simulink model "SPWM_tiaozhi_simscape"  (R2026a)
settings: Solver=ode23t  StartTime=1  StopTime=20  RelTol=1e-5  AbsTol=1e-5
undefined symbols (not defined in the file): PermanentMagnetSynchrono_class
libraries: fl_lib x21, nesl_utility x18, ee_lib x7, eeTransforms x2, elec_conv_HighZElecRef x1, simulink x1
settings Model: SimulationMode=accelerator  Creator=刘炳宏  LastModifiedBy=mushen
settings DebuggingCC: SaveWithParameterizedLinksMsg=none
settings SimscapeCC: SimscapeLogType=none  SimscapeLogDataHistory=5000.0

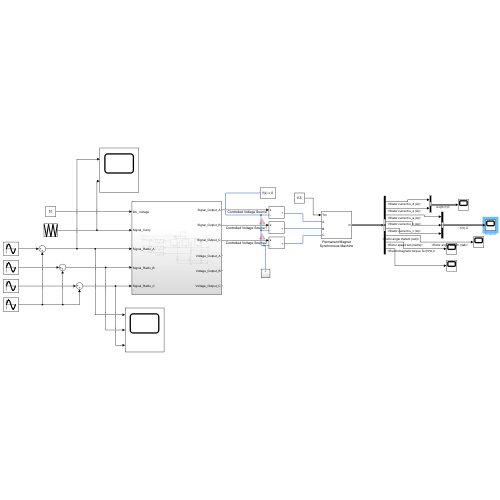
[thumbnail: Simulink's stored preview of the top-level diagram]
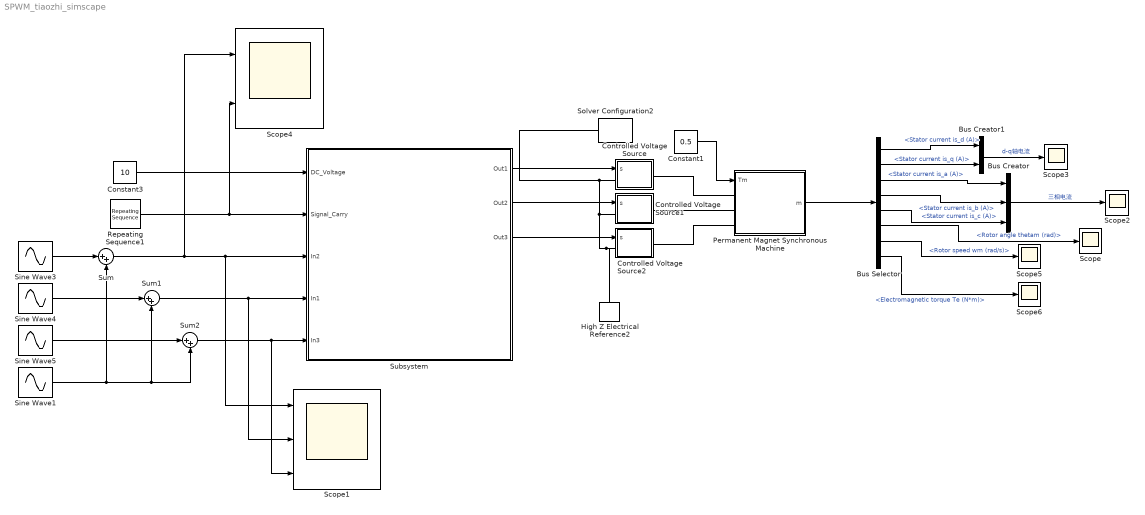
== system SPWM_tiaozhi_simscape ==
  Bus Creator : BusCreator  Inputs=3
  Bus Creator1 : BusCreator  Inputs=2
  Bus Selector : BusSelector  OutputSignals=Stator current is_d (A),Stator current is_q (A),Stator current is_a (A),Stator current is_b (A),Stator current is_c (A),Rotor angle thetam (rad),Rotor speed wm (rad/s),Electromagnetic torque Te (N*m)
  Constant1 : Constant  Value=0.5
  Constant3 : Constant  Value=10
  Controlled Voltage Source : Subsystem
      settings: OpenFcn=elec.conv.unmask(gcb);
  Controlled Voltage Source1 : Subsystem
      settings: OpenFcn=elec.conv.unmask(gcb);
  Controlled Voltage Source2 : Subsystem
      settings: OpenFcn=elec.conv.unmask(gcb);
  High Z Electrical Reference2 : elec_conv_HighZElecRef/High Z Electrical Reference  SystemSampleTime=-1  VariantActivationTime=update diagram  EmptyChoice=off  PassThrough=off  PassThroughVariantControl=(default)  EmptyChoiceVariantControl=(default)  AllowFlexibleInterface=on  Latency=0  AutoFrameSizeCalculation=off
  Permanent Magnet Synchronous Machine : Subsystem
      settings: OpenFcn=elec.conv.unmask(gcb);
  Repeating Sequence1 : simulink/Sources/Repeating Sequence  rep_seq_t=[0,0.5/(5000),1/(5000)]  rep_seq_y=[1,-1,1]
  Scope{,2..3,5..6} (5 alike) : Scope
      Scope settings: ActiveDisplayYMinimum=-0.44345  ActiveDisplayYMaximum=0.09536
      Scope2 settings: ActiveDisplayYMinimum=-3.3210941961077998  ActiveDisplayYMaximum=2.6978662354691325  DataLoggingVariableName=ScopeData2
      Scope3 settings: ActiveDisplayYMinimum=-2.66955  ActiveDisplayYMaximum=3.4348
      Scope5 settings: ActiveDisplayYMinimum=-16.20295  ActiveDisplayYMaximum=14.7299  DataLoggingVariableName=ScopeData3
      Scope6 settings: ActiveDisplayYMinimum=-7.90574  ActiveDisplayYMaximum=7.97374  DataLoggingVariableName=ScopeData4
  Scope1 : Scope  NumInputPorts=3
      settings: SampleTime=0.0000  ActiveDisplayYMinimum=-0.62058705897297939  ActiveDisplayYMaximum=0.62058707725034468  DataLoggingVariableName=Ratio
  Scope4 : Scope  NumInputPorts=2
      settings: SampleTime=0.0000  ActiveDisplayYMinimum=-1.25  ActiveDisplayYMaximum=1.25  DataLoggingVariableName=Ratio1
  Sine Wave1 : Sin  Amplitude=0.02*10  Frequency=6*3.14159*5*10  SampleTime=0
  Sine Wave3 : Sin  Amplitude=0.05*10  Frequency=2*3.14159*5*10  SampleTime=0
  Sine Wave4 : Sin  Amplitude=0.05*10  Frequency=2*3.14159*5*10  Phase=2*3.14159/3  SampleTime=0
  Sine Wave5 : Sin  Amplitude=0.05*10  Frequency=2*3.14159*5*10  Phase=-2*3.14159/3  SampleTime=0
  Solver Configuration2 : nesl_utility/Solver Configuration  PhysicalDomain=network_engine_domain  SubClassName=solver  LeftPortType=input  RightPortType=generic  Tones=[]  Harmonics=[]  SimulateNoise=off  Profile=off  UseLocalSampling=off  EnableSwitchedLinearOptims=on  FrequencyDomain=off  UseCCode=off  RelTol=0.001  AbsTol=0.001  MinStep=1e-09  ToWorkspace=off  RevertToSquareIcSolve=off  NumHomotopyIterations=100  PhasorMode=off  PhasorModeNumHarmonics=1  ConsistencySolver=NEWTON_XTOL_AFTER_FTOL  CanonicalOrdering=UNORDERED  OptimizeIntermediates=UNOPTIMIZED  IndexReductionMethod=DerivativeReplacement  DoDC=off  ResidualTolerance=1e-09  ConsistencyTolSource=GLOBAL  ConsistencyAbsTol=0.001  ConsistencyRelTol=0.001  ConsistencyTolFactor=0.001  UseLocalSolver=off  LocalSolverChoice=NE_BACKWARD_EULER_ADVANCER  ResolveIndetEquations=on  FunctionEvalNumThread=1  LocalSolverSampleTime=0.001  DoFixedCost=off  MaxNonlinIter=3  MaxModeIter=2  ComputeImpulses=off  ImpulseIterations=2  LinearAlgebra=auto  LinearAlgebraNumThread=0  EquationFormulation=NE_TIME_EF  DelaysMemoryBudget=1024  AutomaticFiltering=on  FilteringTimeConstant=0.001  PartitionStorageMethod=AS_NEEDED  PartitionMemoryBudget=1024  PartitionMethod=ROBUST  MultibodyUseLocalSolver=off  MultibodyLocalSolverChoice=ODE1  MultibodyLocalSolverSampleTime=0.001
  Subsystem : Subsystem
  Sum : Sum  Inputs=|++
  Sum1 : Sum  Inputs=|++
  Sum2 : Sum  Inputs=|++
  wires:
  Repeating Sequence1/1 -> Scope4/2, Subsystem/2(Signal_Carry)
  Constant3/1 -> Subsystem/1(DC_Voltage)
  Sine Wave3/1 -> Sum/1
  Sum/1 -> Scope4/1, Scope1/1, Subsystem/3(In2)
  Sum1/1 -> Scope1/2, Subsystem/4(In1)
  Sine Wave4/1 -> Sum1/1
  Sine Wave1/1 -> Sum2/2, Sum1/2, Sum/2
  Sine Wave5/1 -> Sum2/1
  Sum2/1 -> Scope1/3, Subsystem/5(In3)
  Subsystem/1(Out1) -> Controlled Voltage Source/1(s)
  Subsystem/3(Out3) -> Controlled Voltage Source2/1(s)
  Subsystem/2(Out2) -> Controlled Voltage Source1/1(s)
  Bus Selector/5 -> Bus Creator/3  "<Stator current is_c (A)>"
  Bus Selector/4 -> Bus Creator/2  "<Stator current is_b (A)>"
  Bus Selector/2 -> Bus Creator1/2  "<Stator current is_q (A)>"
  Bus Selector/1 -> Bus Creator1/1  "<Stator current is_d (A)>"
  Bus Creator1/1 -> Scope3/1  "d-q轴电流"
  Permanent Magnet Synchronous Machine/1(m) -> Bus Selector/1
  Bus Creator/1 -> Scope2/1  "三相电流"
  Bus Selector/3 -> Bus Creator/1  "<Stator current is_a (A)>"
  Bus Selector/6 -> Scope/1  "<Rotor angle thetam (rad)>"
  Bus Selector/7 -> Scope5/1  "<Rotor speed wm (rad/s)>"
  Bus Selector/8 -> Scope6/1  "<Electromagnetic torque Te (N*m)>"
  Constant1/1 -> Permanent Magnet Synchronous Machine/1(Tm)
  connections:
  Controlled Voltage Source/LConn1 -- Solver Configuration2/RConn1 -- Controlled Voltage Source1/LConn1 -- Controlled Voltage Source2/LConn1 -- High Z Electrical Reference2/LConn1
  Permanent Magnet Synchronous Machine/LConn2 -- Controlled Voltage Source1/RConn1
  Permanent Magnet Synchronous Machine/LConn1 -- Controlled Voltage Source/RConn1
  Permanent Magnet Synchronous Machine/LConn3 -- Controlled Voltage Source2/RConn1

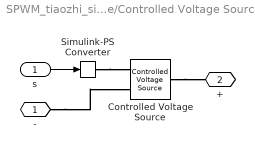
== system SPWM_tiaozhi_simscape/Controlled Voltage Source ==
  s : Inport
  Controlled Voltage Source : fl_lib/Electrical/Electrical Sources/Controlled Voltage Source
  Simulink-PS Converter : nesl_utility/Simulink-PS Converter  PhysicalDomain=network_engine_domain  SubClassName=ps_input  LeftPortType=input  RightPortType=output  PseudoPeriodic=off  Frequencies=[]  NoiseDistribution=none  NoiseParameters=[]  Unit=1  AffineConversion=off  FilteringAndDerivatives=provide  SimscapeFilterOrder=1  InputFilterTimeConstant=0.001  UdotUserProvided=0
  - : PMIOPort  Side=Left
  + : PMIOPort  Port=2  Side=Right
  wires:
  s/1 -> Simulink-PS Converter/1
  connections:
  -/RConn1 -- Controlled Voltage Source/RConn2
  Simulink-PS Converter/RConn1 -- Controlled Voltage Source/RConn1
  Controlled Voltage Source/LConn1 -- +/RConn1

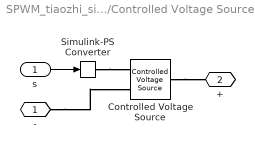
== system SPWM_tiaozhi_simscape/Controlled Voltage Source1 ==
  s : Inport
  Controlled Voltage Source : fl_lib/Electrical/Electrical Sources/Controlled Voltage Source
  Simulink-PS Converter : nesl_utility/Simulink-PS Converter  PhysicalDomain=network_engine_domain  SubClassName=ps_input  LeftPortType=input  RightPortType=output  PseudoPeriodic=off  Frequencies=[]  NoiseDistribution=none  NoiseParameters=[]  Unit=1  AffineConversion=off  FilteringAndDerivatives=provide  SimscapeFilterOrder=1  InputFilterTimeConstant=0.001  UdotUserProvided=0
  - : PMIOPort  Side=Left
  + : PMIOPort  Port=2  Side=Right
  wires:
  s/1 -> Simulink-PS Converter/1
  connections:
  -/RConn1 -- Controlled Voltage Source/RConn2
  Simulink-PS Converter/RConn1 -- Controlled Voltage Source/RConn1
  Controlled Voltage Source/LConn1 -- +/RConn1

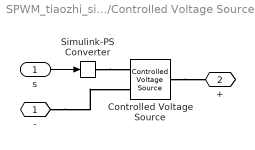
== system SPWM_tiaozhi_simscape/Controlled Voltage Source2 ==
  s : Inport
  Controlled Voltage Source : fl_lib/Electrical/Electrical Sources/Controlled Voltage Source
  Simulink-PS Converter : nesl_utility/Simulink-PS Converter  PhysicalDomain=network_engine_domain  SubClassName=ps_input  LeftPortType=input  RightPortType=output  PseudoPeriodic=off  Frequencies=[]  NoiseDistribution=none  NoiseParameters=[]  Unit=1  AffineConversion=off  FilteringAndDerivatives=provide  SimscapeFilterOrder=1  InputFilterTimeConstant=0.001  UdotUserProvided=0
  - : PMIOPort  Side=Left
  + : PMIOPort  Port=2  Side=Right
  wires:
  s/1 -> Simulink-PS Converter/1
  connections:
  -/RConn1 -- Controlled Voltage Source/RConn2
  Simulink-PS Converter/RConn1 -- Controlled Voltage Source/RConn1
  Controlled Voltage Source/LConn1 -- +/RConn1

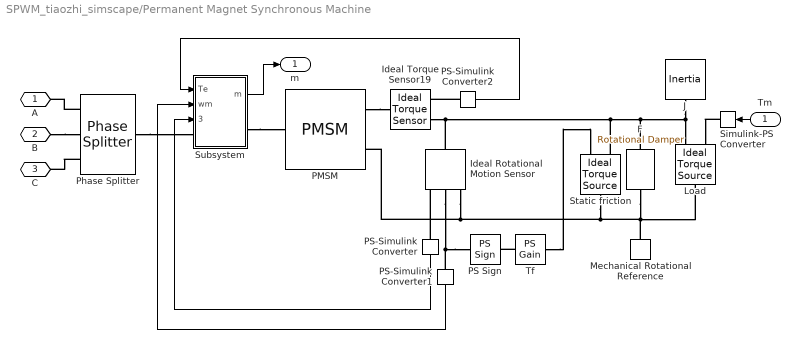
== system SPWM_tiaozhi_simscape/Permanent Magnet Synchronous Machine ==
  Tm : Inport
  F : fl_lib/Mechanical/Rotational Elements/Rotational Damper  D=0.0003505 N*m/(rad/s)  w_specify=on  w_priority=High  w=0 rad/s  w_nominal_specify=off  w_nominal_value=1  w_nominal_unit=rad/s  t_specify=off  t_priority=None  t=0 N*m  t_nominal_specify=off  t_nominal_value=1  t_nominal_unit=N*m
  Ideal Rotational Motion Sensor : fl_lib/Mechanical/Mechanical Sensors/Ideal Rotational Motion Sensor  reference=foundation.enum.MeasurementReference.difference  acceleration_port=false  velocity_port=true  position_port=true  wrap_angle=simscape.enum.onoff.off  offset=1 deg
  Ideal Torque Sensor19 : fl_lib/Mechanical/Mechanical Sensors/Ideal Torque Sensor
  J : fl_lib/Mechanical/Rotational Elements/Inertia  inertia=0.00062 kg*m^2  num_ports=foundation.enum.numPorts2.one  w_specify=on  w_priority=High  w=0 rad/s  w_nominal_specify=off  w_nominal_value=1  w_nominal_unit=rad/s  t_specify=off  t_priority=None  t=0 N*m  t_nominal_specify=off  t_nominal_value=1  t_nominal_unit=N*m
  Load : fl_lib/Mechanical/Mechanical Sources/Ideal Torque Source
  Mechanical Rotational Reference : fl_lib/Mechanical/Rotational Elements/Mechanical Rotational Reference
  PMSM : ee_lib/Electromechanical/Permanent Magnet/PMSM  port_option=ee.enum.threePhasePort.composite  winding_type=ee.enum.statorconnection.wye  machine_param=ee.enum.pmsm.parameterization.constant  nPolePairs=10  pmflux_param=1  pm_flux_linkage=PermanentMagnetSynchrono_class('Torque Tm',[0.00062 0.0003505 10 0],4,'Flux linkage established by magnets (V.s)',0.074147,134.4878,1.1122,'Aligned with phase A axis (original Park)',[0 1 0 0],'Sinusoidal',120,'3',[0 0 0 0 0 0]).objParamMappingDerived.NewDerivedParam.pm_flux_linkage Wb  torque_constant=0.18 N*m/A  back_emf_constant=0.18 V/(rad/s)  stator_param=1  Ld=0.0085 H  Lq=0.0085 H  idVec=[-200, 0, 200] A  iqVec=[-200, 0, 200] A  LdMatrix=0.0002 * ones(3, 3) H  LqMatrix=0.0002 * ones(3, 3) H  PmMatrix=0.1 * ones(3, 3) Wb  ktMatrix=0.18 * ones(3, 3) N*m/A  keMatrix=0.18 * ones(3, 3) V/(rad/s)  L0=1e-09 H  Ls=0.0002 H  Lm=-0.00002 H  Ms=0.00002 H  Rs=0.18 Ohm  zero_sequence=0  axes_param=2  loss_param=ee.enum.ironloss.none  losses_oc=[0, 0, 0] W  losses_sc=[0, 0, 0] W  f_losses=60 Hz  Isc_losses=95 A  J=0 kg*m^2  lam=0 N*m/(rad/s)  i_d_specify=on  i_d_priority=High  i_d=PermanentMagnetSynchrono_class('Torque Tm',[0.00062 0.0003505 10 0],4,'Flux linkage established by magnets (V.s)',0.074147,134.4878,1.1122,'Aligned with phase A axis (original Park)',[0 1 0 0],'Sinusoidal',120,'3',[0 0 0 0 0 0]).objParamMappingDerived.NewDerivedParam.i_d A  i_d_nominal_specify=off  i_d_nominal_value=1  i_d_nominal_unit=A  i_q_specify=on  i_q_priority=High  i_q=PermanentMagnetSynchrono_class('Torque Tm',[0.00062 0.0003505 10 0],4,'Flux linkage established by magnets (V.s)',0.074147,134.4878,1.1122,'Aligned with phase A axis (original Park)',[0 1 0 0],'Sinusoidal',120,'3',[0 0 0 0 0 0]).objParamMappingDerived.NewDerivedParam.i_q A  i_q_nominal_specify=off  i_q_nominal_value=1  i_q_nominal_unit=A  torque_specify=off  torque_priority=None  torque=0 N*m  torque_nominal_specify=off  torque_nominal_value=1  torque_nominal_unit=N*m  angular_velocity_specify=on  angular_velocity_priority=High  angular_velocity=0 rad/s  angular_velocity_nominal_specify=off  angular_velocity_nominal_value=1  angular_velocity_nominal_unit=rpm  angular_position_specify=on  angular_position_priority=High  angular_position=1 deg  angular_position_nominal_specify=off  angular_position_nominal_value=1  angular_position_nominal_unit=deg  alpha=3.93e-3 1/K  alpha_flux=-0.001 1/K  Tmeas=298.15 K  stator_thermal_mass=100 J/K  rotor_thermal_mass=200 J/K  Rm_percent_rotor=90  Rd_percent_rotor=30  temperatureA_specify=off  temperatureA_priority=High  temperatureA=25 degC  temperatureA_nominal_specify=off  temperatureA_nominal_value=1  temperatureA_nominal_unit=degC  temperatureB_specify=off  temperatureB_priority=High  temperatureB=25 degC  temperatureB_nominal_specify=off  temperatureB_nominal_value=1  temperatureB_nominal_unit=degC  temperatureC_specify=off  temperatureC_priority=High  temperatureC=25 degC  temperatureC_nominal_specify=off  temperatureC_nominal_value=1  temperatureC_nominal_unit=degC  temperatureR_specify=off  temperatureR_priority=High  temperatureR=25 degC  temperatureR_nominal_specify=off  temperatureR_nominal_value=1  temperatureR_nominal_unit=degC
  PS Sign : fl_lib/Physical Signals/Nonlinear Operators/PS Sign
  PS-Simulink Converter : nesl_utility/PS-Simulink Converter  PhysicalDomain=network_engine_domain  SubClassName=ps_output  LeftPortType=input  RightPortType=output  PseudoPeriodic=off  Frequencies=[]  VectorFormat=1-D array  Unit=1  AffineConversion=off
  PS-Simulink Converter1 : nesl_utility/PS-Simulink Converter  PhysicalDomain=network_engine_domain  SubClassName=ps_output  LeftPortType=input  RightPortType=output  PseudoPeriodic=off  Frequencies=[]  VectorFormat=1-D array  Unit=1  AffineConversion=off
  PS-Simulink Converter2 : nesl_utility/PS-Simulink Converter  PhysicalDomain=network_engine_domain  SubClassName=ps_output  LeftPortType=input  RightPortType=output  PseudoPeriodic=off  Frequencies=[]  VectorFormat=1-D array  Unit=1  AffineConversion=off
  Phase Splitter : ee_lib/Connectors & References/Phase Splitter
  Simulink-PS Converter : nesl_utility/Simulink-PS Converter  PhysicalDomain=network_engine_domain  SubClassName=ps_input  LeftPortType=input  RightPortType=output  PseudoPeriodic=off  Frequencies=[]  NoiseDistribution=none  NoiseParameters=[]  Unit=1  AffineConversion=off  FilteringAndDerivatives=provide  SimscapeFilterOrder=1  InputFilterTimeConstant=0.001  UdotUserProvided=0
  Static friction : fl_lib/Mechanical/Mechanical Sources/Ideal Torque Source
  Subsystem : Subsystem
  Tf : fl_lib/Physical Signals/Functions/PS Gain  gain=PermanentMagnetSynchrono_class('Torque Tm',[0.00062 0.0003505 10 0],4,'Flux linkage established by magnets (V.s)',0.074147,134.4878,1.1122,'Aligned with phase A axis (original Park)',[0 1 0 0],'Sinusoidal',120,'3',[0 0 0 0 0 0]).objParamMappingDerived.NewDerivedParam.Tf
  A : PMIOPort  Side=Left
  B : PMIOPort  Port=2  Side=Left
  C : PMIOPort  Port=3  Side=Left
  m : Outport  VectorParamsAs1DForOutWhenUnconnected=off
  wires:
  PS-Simulink Converter1/1 -> Subsystem/2(wm)
  PS-Simulink Converter/1 -> Subsystem/3(thetam)
  PS-Simulink Converter2/1 -> Subsystem/1(Te)
  Subsystem/1(m) -> m/1
  Tm/1 -> Simulink-PS Converter/1
  connections:
  PS-Simulink Converter2/LConn1 -- Ideal Torque Sensor19/RConn2
  Phase Splitter/LConn1 -- Subsystem/LConn1
  Subsystem/RConn1 -- PMSM/LConn1
  PS-Simulink Converter/LConn1 -- Ideal Rotational Motion Sensor/RConn3
  Tf/RConn1 -- Static friction/RConn1
  PS Sign/LConn1 -- PS-Simulink Converter1/LConn1 -- Ideal Rotational Motion Sensor/RConn2
  Tf/LConn1 -- PS Sign/RConn1
  PMSM/RConn1 -- Ideal Torque Sensor19/LConn1
  Ideal Torque Sensor19/RConn1 -- Static friction/RConn2 -- F/LConn1 -- Load/RConn2 -- J/LConn1 -- Ideal Rotational Motion Sensor/LConn1
  Phase Splitter/RConn3 -- C/RConn1
  Phase Splitter/RConn1 -- A/RConn1
  B/RConn1 -- Phase Splitter/RConn2
  Simulink-PS Converter/RConn1 -- Load/RConn1
  Load/LConn1 -- F/RConn1 -- Static friction/LConn1 -- PMSM/RConn2 -- Ideal Rotational Motion Sensor/RConn1 -- Mechanical Rotational Reference/LConn1

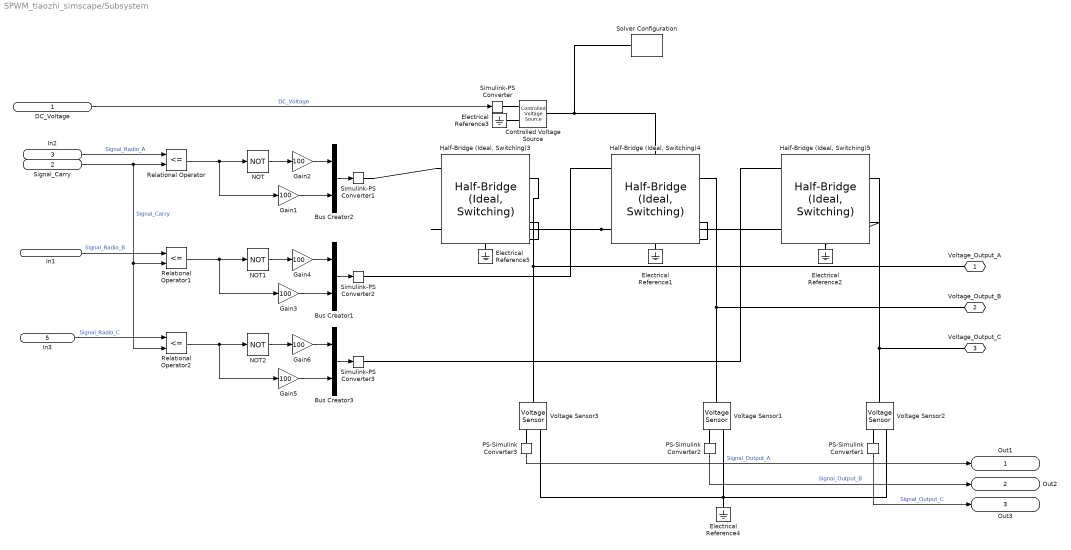
== system SPWM_tiaozhi_simscape/Subsystem ==
  DC_Voltage : Inport
  Signal_Carry : Inport  Port=2
  In2 : Inport  Port=3
  In1 : Inport  Port=4
  In3 : Inport  Port=5
  Bus Creator1 : BusCreator  Inputs=2
  Bus Creator2 : BusCreator  Inputs=2
  Bus Creator3 : BusCreator  Inputs=2
  Controlled Voltage Source : fl_lib/Electrical/Electrical Sources/Controlled Voltage Source
  Electrical Reference{1..5} (5 alike) : fl_lib/Electrical/Electrical Elements/Electrical Reference
  Gain{1..6} (6 alike) : Gain  Gain=100  OutDataTypeStr=double
  "Half-Bridge (Ideal, Switching)3" : ee_lib/Semiconductors & Converters/Half-Bridge (Ideal, Switching)  control_port=ee.enum.controlport.ps  device_type=ee.enum.converters.switches.mosfet  gto_Vgt=6 V  gto_Vgt_off=-1 V  gto_Ih=1 A  gto_thermal_loss_option=ee.enum.converters.thermalLossOption.constantvalues  gto_Vf=0.8 V  gto_Ron=0.001 Ohm  gto_Von_data=[0, .1, .6, .8, 1, 1.3, 1.6, 2, 2.4; 0, .1, .7, 1, 1.2, 1.5, 1.9, 2.4, 2.8] V  gto_Tj=[298.15, 398.15] K  gto_Iout_data=[0, .1, 1, 5, 10, 20, 40, 70, 100] A  igbt_Vth=6 V  igbt_thermal_loss_option=ee.enum.converters.thermalLossOption.constantvalues  igbt_Vf=0.8 V  igbt_Ron=0.001 Ohm  igbt_Von_data=[0, .1, .6, .8, 1, 1.3, 1.6, 2, 2.4; 0, .1, .7, 1, 1.2, 1.5, 1.9, 2.4, 2.8] V  igbt_Tj=[298.15, 398.15] K  igbt_Iout_data=[0, .1, 1, 5, 10, 20, 40, 70, 100] A  mosfet_Vth=2 V  mosfet_thermal_loss_option=ee.enum.converters.thermalLossOption.constantvalues  mosfet_Rds=0.01 Ohm  mosfet_Von_data=[0, 1.1, 1.3, 1.45, 1.75, 2.25, 2.7; 0, 1, 1.15, 1.35, 1.7, 2.35, 3] V  mosfet_Tj=[298.15, 398.15] K  mosfet_Iout_data=[0, 10, 50, 100, 200, 400, 600] A  Goff=1e-6 1/Ohm  separateAxesForDiodeErec=false  igbt_tabulateWithVce=false  mosfet_tabulateWithVds=false  gto_Eon_data=[0, .0024, .024, .12, .2, .48, 1.04, 2.16, 3.24; 0, .003, .03, .15, .25, .6, 1.3, 2.7, 4.05] * 1e-3 J  igbt_Eon_data=[0, .0024, .024, .12, .2, .48, 1.04, 2.16, 3.24; 0, .003, .03, .15, .25, .6, 1.3, 2.7, 4.05] * 1e-3 J  mosfet_Eon_data=[0, .29, 1.43, 2.86, 5.71, 13.14, 22.86; 0, .57, 2.63, 5.14, 10.29, 20.57, 30.29] * 1e-3 J  gto_Eoff_data=[0, .0007, .0066, .033, .066, .17, .33, .83, 1.5; 0, .001, .01, .05, .1, .25, .5, 1.2, 2.2] * 1e-3 J  igbt_Eoff_data=[0, .0007, .0066, .033, .066, .17, .33, .83, 1.5; 0, .001, .01, .05, .1, .25, .5, 1.2, 2.2] * 1e-3 J  mosfet_Eoff_data=[0, .21, 1.07, 2.14, 4.29, 9.86, 17.14; 0, .43, 1.97, 3.86, 7.71, 15.43, 22.71] * 1e-3 J  igbt_Eon_data_3D=[zeros(2, 9, 3)] J  mosfet_Eon_data_3D=[zeros(2, 7, 3)] J  igbt_Eoff_data_3D=[zeros(2, 9, 3)] J  mosfet_Eoff_data_3D=[zeros(2, 7, 3)] J  gto_Erec_data=[0, .0031, .021, .11, .21, .43, .99, 1.71, 3.078; 0, .0041, .043, .2, .39, .77, 1.54, 2.27, 4.08] * 1e-3 J  igbt_Erec_data=[0, .0031, .021, .11, .21, .43, .99, 1.71, 3.078; 0, .0041, .043, .2, .39, .77, 1.54, 2.27, 4.08] * 1e-3 J  mosfet_Erec_data=[0, .0031, .021, .11, .21, .43, .99; 0, .0041, .043, .2, .39, .77, 1.54] * 1e-3 J  gto_Tj_loss=[298.15, 398.15] K  igbt_Tj_loss=[298.15, 398.15] K  mosfet_Tj_loss=[298.15, 398.15] K  gto_Iout_data_loss=[0, .1, 1, 5, 10, 20, 40, 70, 100] A  igbt_Iout_data_loss=[0, .1, 1, 5, 10, 20, 40, 70, 100] A  mosfet_Iout_data_loss=[0, 10, 50, 100, 200, 400, 600] A  gto_Eon_scalar=22.86e-3 J  igbt_Eon_scalar=22.86e-3 J  mosfet_Eon_scalar=22.86e-3 J  gto_Eoff_scalar=17.14e-3 J  igbt_Eoff_scalar=17.14e-3 J  mosfet_Eoff_scalar=17.14e-3 J  gto_Erec_scalar=5.70e-3 J  igbt_Erec_scalar=5.70e-3 J  mosfet_Erec_scalar=5.70e-3 J  gto_Iout_scalar=600 A  igbt_Iout_scalar=600 A  mosfet_Iout_scalar=600 A  igbt_Vce_loss=[0, 150, 300] V  mosfet_Vds_loss=[0, 150, 300] V  Voff=300 V  gtoDiodeErecMat3D=zeros(2, 3, 3) J  igbtDiodeErecMat3D=zeros(2, 3, 3) J  mosfetDiodeErecMat3D=zeros(2, 3, 3) J  gtoTjVecForErec=[298.15, 398.15] K  igbtTjVecForErec=[298.15, 398.15] K  mosfetTjVecForErec=[298.15, 398.15] K  gtoIakVecForErec=[0, 20, 40] A  igbtIceVecForErec=[0, 20, 40] A  mosfetIdsVecForErec=[0, 100, 200] A  gtoVakVecForErec=[0, 150, 300] V  igbtVceVecForErec=[0, 150, 300] V  mosfetVdsVecForErec=[0, 150, 300] V  gto_Eoff_natural_commutation=10e-3 J  applySwLossToSupply=false  tauApplySwLoss=1e-3 s  diode_param=ee.enum.include.yes  diode_ModelType=ee.enum.converters.diodeModelType.pwl  diode_TableType=ee.enum.diode.tableType.IfMat  diode_ReverseIVType=ee.enum.diode.diodeReverseIV.constant  diode_IfMat=[.07, .12, .19, 1.75, 4.24, 7.32, 11.2; .16, .3, .72, 2.14, 4.02, 6.35, 9.12] A  diode_VfMat=[.9, 1.15, 1.25, 1.5, 1.75, 2.17, 2.6, 2.85; .58, .68, .75, 1.1, 1.38, 1.77, 2.27, 2.7] V  diode_TjVec=[25, 125] degC  diode_VfVec=[.5, .7, .9, 1.3, 1.7, 2.1, 2.5] V  diode_IfVec=[.1, .2, .5, 1, 2, 4, 7, 10] A  diode_IrMat=[1e-06, 2e-06, 5e-06, 1e-05, 2.5e-05, 5e-05, .0001; 2e-06, 5e-06, 1e-05, 4e-05, 8e-05, .0002, .0005] A  diode_VrMat=[10, 100, 200, 250, 300, 325, 350; 10, 70, 160, 220, 270, 300, 320] V  diode_VrVec=[10, 20, 40, 50, 70, 80, 100] V  diode_IrVec=[1e-06, 2e-06, 5e-06, 1e-05, 2e-05, 5e-05, .0001] A  diode_Vf=0.8 V  diode_Ron=0.001 Ohm  diode_Goff=1e-5 1/Ohm  separateThermalPort=false  separateThermalPortsForDiodes=false  thermal_network_parameterization=ee.enum.thermalNetworkTopology.external  thermal_mass_parameterization=ee.enum.thermalNetwork.timeconstant  Rth=[.03, .2] K/W  Rth_Cauer=[.03, .1, .2] K/W  Rth_Foster=[.08, .14, .22, .16] K/W  thermal_mass=[3, 25] J/K  thermal_mass_Cauer=[3, 10, 25] J/K  thermal_mass_Foster=[.001, .005, .05, .5] J/K  thermal_time_constant=[.1, 5] s  thermal_time_constant_Cauer=[.1, 1, 5] s  thermal_time_constant_Foster=[7e-05, .0007, .01, .08] s  thermal_mass_initial_temperatures=[25, 25] degC  thermal_mass_initial_temperatures_Cauer=[25, 25, 25] degC  junction_thermal_mass=0.1 J/K  Tvec_initial_Foster=[25, 25, 25, 25] degC  RthDiode=[.03, .2] K/W  RthCauerDiode=[.03, .1, .2] K/W  RthFosterDiode=[.08, .14, .22, .16] K/W  ThermalMassDiode=[3, 25] J/K  ThermalMassCauerDiode=[3, 10, 25] J/K  ThermalMassFosterDiode=[.001, .005, .05, .5] J/K  ThermalTauDiode=[.1, 5] s  ThermalTauCauerDiode=[.1, 1, 5] s  ThermalTauFosterDiode=[7e-05, .0007, .01, .08] s  ThermalMassInitTempDiode=[25, 25] degC  ThermalMassInitTempCauerDiode=[25, 25, 25] degC  JunctionThermalMassDiode=0.1 J/K  TVecInitialFosterDiode=[25, 25, 25, 25] degC  junction_temperature_specify=off  junction_temperature_priority=None  junction_temperature=25 degC  junction_temperature_nominal_specify=off  junction_temperature_nominal_value=1  junction_temperature_nominal_unit=degC  upperSwitchTemp_specify=off  upperSwitchTemp_priority=None  upperSwitchTemp=25 degC  upperSwitchTemp_nominal_specify=off  upperSwitchTemp_nominal_value=1  upperSwitchTemp_nominal_unit=degC  lowerSwitchTemp_specify=off  lowerSwitchTemp_priority=None  lowerSwitchTemp=25 degC  lowerSwitchTemp_nominal_specify=off  lowerSwitchTemp_nominal_value=1  lowerSwitchTemp_nominal_unit=degC  upperDiodeTemp_specify=off  upperDiodeTemp_priority=None  upperDiodeTemp=25 degC  upperDiodeTemp_nominal_specify=off  upperDiodeTemp_nominal_value=1  upperDiodeTemp_nominal_unit=degC  lowerDiodeTemp_specify=off  lowerDiodeTemp_priority=None  lowerDiodeTemp=25 degC  lowerDiodeTemp_nominal_specify=off  lowerDiodeTemp_nominal_value=1  lowerDiodeTemp_nominal_unit=degC
  "Half-Bridge (Ideal, Switching)4" : ee_lib/Semiconductors & Converters/Half-Bridge (Ideal, Switching)  control_port=ee.enum.controlport.ps  device_type=ee.enum.converters.switches.mosfet  gto_Vgt=6 V  gto_Vgt_off=-1 V  gto_Ih=1 A  gto_thermal_loss_option=ee.enum.converters.thermalLossOption.constantvalues  gto_Vf=0.8 V  gto_Ron=0.001 Ohm  gto_Von_data=[0, .1, .6, .8, 1, 1.3, 1.6, 2, 2.4; 0, .1, .7, 1, 1.2, 1.5, 1.9, 2.4, 2.8] V  gto_Tj=[298.15, 398.15] K  gto_Iout_data=[0, .1, 1, 5, 10, 20, 40, 70, 100] A  igbt_Vth=6 V  igbt_thermal_loss_option=ee.enum.converters.thermalLossOption.constantvalues  igbt_Vf=0.8 V  igbt_Ron=0.001 Ohm  igbt_Von_data=[0, .1, .6, .8, 1, 1.3, 1.6, 2, 2.4; 0, .1, .7, 1, 1.2, 1.5, 1.9, 2.4, 2.8] V  igbt_Tj=[298.15, 398.15] K  igbt_Iout_data=[0, .1, 1, 5, 10, 20, 40, 70, 100] A  mosfet_Vth=2 V  mosfet_thermal_loss_option=ee.enum.converters.thermalLossOption.constantvalues  mosfet_Rds=0.01 Ohm  mosfet_Von_data=[0, 1.1, 1.3, 1.45, 1.75, 2.25, 2.7; 0, 1, 1.15, 1.35, 1.7, 2.35, 3] V  mosfet_Tj=[298.15, 398.15] K  mosfet_Iout_data=[0, 10, 50, 100, 200, 400, 600] A  Goff=1e-6 1/Ohm  separateAxesForDiodeErec=false  igbt_tabulateWithVce=false  mosfet_tabulateWithVds=false  gto_Eon_data=[0, .0024, .024, .12, .2, .48, 1.04, 2.16, 3.24; 0, .003, .03, .15, .25, .6, 1.3, 2.7, 4.05] * 1e-3 J  igbt_Eon_data=[0, .0024, .024, .12, .2, .48, 1.04, 2.16, 3.24; 0, .003, .03, .15, .25, .6, 1.3, 2.7, 4.05] * 1e-3 J  mosfet_Eon_data=[0, .29, 1.43, 2.86, 5.71, 13.14, 22.86; 0, .57, 2.63, 5.14, 10.29, 20.57, 30.29] * 1e-3 J  gto_Eoff_data=[0, .0007, .0066, .033, .066, .17, .33, .83, 1.5; 0, .001, .01, .05, .1, .25, .5, 1.2, 2.2] * 1e-3 J  igbt_Eoff_data=[0, .0007, .0066, .033, .066, .17, .33, .83, 1.5; 0, .001, .01, .05, .1, .25, .5, 1.2, 2.2] * 1e-3 J  mosfet_Eoff_data=[0, .21, 1.07, 2.14, 4.29, 9.86, 17.14; 0, .43, 1.97, 3.86, 7.71, 15.43, 22.71] * 1e-3 J  igbt_Eon_data_3D=[zeros(2, 9, 3)] J  mosfet_Eon_data_3D=[zeros(2, 7, 3)] J  igbt_Eoff_data_3D=[zeros(2, 9, 3)] J  mosfet_Eoff_data_3D=[zeros(2, 7, 3)] J  gto_Erec_data=[0, .0031, .021, .11, .21, .43, .99, 1.71, 3.078; 0, .0041, .043, .2, .39, .77, 1.54, 2.27, 4.08] * 1e-3 J  igbt_Erec_data=[0, .0031, .021, .11, .21, .43, .99, 1.71, 3.078; 0, .0041, .043, .2, .39, .77, 1.54, 2.27, 4.08] * 1e-3 J  mosfet_Erec_data=[0, .0031, .021, .11, .21, .43, .99; 0, .0041, .043, .2, .39, .77, 1.54] * 1e-3 J  gto_Tj_loss=[298.15, 398.15] K  igbt_Tj_loss=[298.15, 398.15] K  mosfet_Tj_loss=[298.15, 398.15] K  gto_Iout_data_loss=[0, .1, 1, 5, 10, 20, 40, 70, 100] A  igbt_Iout_data_loss=[0, .1, 1, 5, 10, 20, 40, 70, 100] A  mosfet_Iout_data_loss=[0, 10, 50, 100, 200, 400, 600] A  gto_Eon_scalar=22.86e-3 J  igbt_Eon_scalar=22.86e-3 J  mosfet_Eon_scalar=22.86e-3 J  gto_Eoff_scalar=17.14e-3 J  igbt_Eoff_scalar=17.14e-3 J  mosfet_Eoff_scalar=17.14e-3 J  gto_Erec_scalar=5.70e-3 J  igbt_Erec_scalar=5.70e-3 J  mosfet_Erec_scalar=5.70e-3 J  gto_Iout_scalar=600 A  igbt_Iout_scalar=600 A  mosfet_Iout_scalar=600 A  igbt_Vce_loss=[0, 150, 300] V  mosfet_Vds_loss=[0, 150, 300] V  Voff=300 V  gtoDiodeErecMat3D=zeros(2, 3, 3) J  igbtDiodeErecMat3D=zeros(2, 3, 3) J  mosfetDiodeErecMat3D=zeros(2, 3, 3) J  gtoTjVecForErec=[298.15, 398.15] K  igbtTjVecForErec=[298.15, 398.15] K  mosfetTjVecForErec=[298.15, 398.15] K  gtoIakVecForErec=[0, 20, 40] A  igbtIceVecForErec=[0, 20, 40] A  mosfetIdsVecForErec=[0, 100, 200] A  gtoVakVecForErec=[0, 150, 300] V  igbtVceVecForErec=[0, 150, 300] V  mosfetVdsVecForErec=[0, 150, 300] V  gto_Eoff_natural_commutation=10e-3 J  applySwLossToSupply=false  tauApplySwLoss=1e-3 s  diode_param=ee.enum.include.yes  diode_ModelType=ee.enum.converters.diodeModelType.pwl  diode_TableType=ee.enum.diode.tableType.IfMat  diode_ReverseIVType=ee.enum.diode.diodeReverseIV.constant  diode_IfMat=[.07, .12, .19, 1.75, 4.24, 7.32, 11.2; .16, .3, .72, 2.14, 4.02, 6.35, 9.12] A  diode_VfMat=[.9, 1.15, 1.25, 1.5, 1.75, 2.17, 2.6, 2.85; .58, .68, .75, 1.1, 1.38, 1.77, 2.27, 2.7] V  diode_TjVec=[25, 125] degC  diode_VfVec=[.5, .7, .9, 1.3, 1.7, 2.1, 2.5] V  diode_IfVec=[.1, .2, .5, 1, 2, 4, 7, 10] A  diode_IrMat=[1e-06, 2e-06, 5e-06, 1e-05, 2.5e-05, 5e-05, .0001; 2e-06, 5e-06, 1e-05, 4e-05, 8e-05, .0002, .0005] A  diode_VrMat=[10, 100, 200, 250, 300, 325, 350; 10, 70, 160, 220, 270, 300, 320] V  diode_VrVec=[10, 20, 40, 50, 70, 80, 100] V  diode_IrVec=[1e-06, 2e-06, 5e-06, 1e-05, 2e-05, 5e-05, .0001] A  diode_Vf=0.8 V  diode_Ron=0.001 Ohm  diode_Goff=1e-5 1/Ohm  separateThermalPort=false  separateThermalPortsForDiodes=false  thermal_network_parameterization=ee.enum.thermalNetworkTopology.external  thermal_mass_parameterization=ee.enum.thermalNetwork.timeconstant  Rth=[.03, .2] K/W  Rth_Cauer=[.03, .1, .2] K/W  Rth_Foster=[.08, .14, .22, .16] K/W  thermal_mass=[3, 25] J/K  thermal_mass_Cauer=[3, 10, 25] J/K  thermal_mass_Foster=[.001, .005, .05, .5] J/K  thermal_time_constant=[.1, 5] s  thermal_time_constant_Cauer=[.1, 1, 5] s  thermal_time_constant_Foster=[7e-05, .0007, .01, .08] s  thermal_mass_initial_temperatures=[25, 25] degC  thermal_mass_initial_temperatures_Cauer=[25, 25, 25] degC  junction_thermal_mass=0.1 J/K  Tvec_initial_Foster=[25, 25, 25, 25] degC  RthDiode=[.03, .2] K/W  RthCauerDiode=[.03, .1, .2] K/W  RthFosterDiode=[.08, .14, .22, .16] K/W  ThermalMassDiode=[3, 25] J/K  ThermalMassCauerDiode=[3, 10, 25] J/K  ThermalMassFosterDiode=[.001, .005, .05, .5] J/K  ThermalTauDiode=[.1, 5] s  ThermalTauCauerDiode=[.1, 1, 5] s  ThermalTauFosterDiode=[7e-05, .0007, .01, .08] s  ThermalMassInitTempDiode=[25, 25] degC  ThermalMassInitTempCauerDiode=[25, 25, 25] degC  JunctionThermalMassDiode=0.1 J/K  TVecInitialFosterDiode=[25, 25, 25, 25] degC  junction_temperature_specify=off  junction_temperature_priority=None  junction_temperature=25 degC  junction_temperature_nominal_specify=off  junction_temperature_nominal_value=1  junction_temperature_nominal_unit=degC  upperSwitchTemp_specify=off  upperSwitchTemp_priority=None  upperSwitchTemp=25 degC  upperSwitchTemp_nominal_specify=off  upperSwitchTemp_nominal_value=1  upperSwitchTemp_nominal_unit=degC  lowerSwitchTemp_specify=off  lowerSwitchTemp_priority=None  lowerSwitchTemp=25 degC  lowerSwitchTemp_nominal_specify=off  lowerSwitchTemp_nominal_value=1  lowerSwitchTemp_nominal_unit=degC  upperDiodeTemp_specify=off  upperDiodeTemp_priority=None  upperDiodeTemp=25 degC  upperDiodeTemp_nominal_specify=off  upperDiodeTemp_nominal_value=1  upperDiodeTemp_nominal_unit=degC  lowerDiodeTemp_specify=off  lowerDiodeTemp_priority=None  lowerDiodeTemp=25 degC  lowerDiodeTemp_nominal_specify=off  lowerDiodeTemp_nominal_value=1  lowerDiodeTemp_nominal_unit=degC
  "Half-Bridge (Ideal, Switching)5" : ee_lib/Semiconductors & Converters/Half-Bridge (Ideal, Switching)  control_port=ee.enum.controlport.ps  device_type=ee.enum.converters.switches.mosfet  gto_Vgt=6 V  gto_Vgt_off=-1 V  gto_Ih=1 A  gto_thermal_loss_option=ee.enum.converters.thermalLossOption.constantvalues  gto_Vf=0.8 V  gto_Ron=0.001 Ohm  gto_Von_data=[0, .1, .6, .8, 1, 1.3, 1.6, 2, 2.4; 0, .1, .7, 1, 1.2, 1.5, 1.9, 2.4, 2.8] V  gto_Tj=[298.15, 398.15] K  gto_Iout_data=[0, .1, 1, 5, 10, 20, 40, 70, 100] A  igbt_Vth=6 V  igbt_thermal_loss_option=ee.enum.converters.thermalLossOption.constantvalues  igbt_Vf=0.8 V  igbt_Ron=0.001 Ohm  igbt_Von_data=[0, .1, .6, .8, 1, 1.3, 1.6, 2, 2.4; 0, .1, .7, 1, 1.2, 1.5, 1.9, 2.4, 2.8] V  igbt_Tj=[298.15, 398.15] K  igbt_Iout_data=[0, .1, 1, 5, 10, 20, 40, 70, 100] A  mosfet_Vth=2 V  mosfet_thermal_loss_option=ee.enum.converters.thermalLossOption.constantvalues  mosfet_Rds=0.01 Ohm  mosfet_Von_data=[0, 1.1, 1.3, 1.45, 1.75, 2.25, 2.7; 0, 1, 1.15, 1.35, 1.7, 2.35, 3] V  mosfet_Tj=[298.15, 398.15] K  mosfet_Iout_data=[0, 10, 50, 100, 200, 400, 600] A  Goff=1e-6 1/Ohm  separateAxesForDiodeErec=false  igbt_tabulateWithVce=false  mosfet_tabulateWithVds=false  gto_Eon_data=[0, .0024, .024, .12, .2, .48, 1.04, 2.16, 3.24; 0, .003, .03, .15, .25, .6, 1.3, 2.7, 4.05] * 1e-3 J  igbt_Eon_data=[0, .0024, .024, .12, .2, .48, 1.04, 2.16, 3.24; 0, .003, .03, .15, .25, .6, 1.3, 2.7, 4.05] * 1e-3 J  mosfet_Eon_data=[0, .29, 1.43, 2.86, 5.71, 13.14, 22.86; 0, .57, 2.63, 5.14, 10.29, 20.57, 30.29] * 1e-3 J  gto_Eoff_data=[0, .0007, .0066, .033, .066, .17, .33, .83, 1.5; 0, .001, .01, .05, .1, .25, .5, 1.2, 2.2] * 1e-3 J  igbt_Eoff_data=[0, .0007, .0066, .033, .066, .17, .33, .83, 1.5; 0, .001, .01, .05, .1, .25, .5, 1.2, 2.2] * 1e-3 J  mosfet_Eoff_data=[0, .21, 1.07, 2.14, 4.29, 9.86, 17.14; 0, .43, 1.97, 3.86, 7.71, 15.43, 22.71] * 1e-3 J  igbt_Eon_data_3D=[zeros(2, 9, 3)] J  mosfet_Eon_data_3D=[zeros(2, 7, 3)] J  igbt_Eoff_data_3D=[zeros(2, 9, 3)] J  mosfet_Eoff_data_3D=[zeros(2, 7, 3)] J  gto_Erec_data=[0, .0031, .021, .11, .21, .43, .99, 1.71, 3.078; 0, .0041, .043, .2, .39, .77, 1.54, 2.27, 4.08] * 1e-3 J  igbt_Erec_data=[0, .0031, .021, .11, .21, .43, .99, 1.71, 3.078; 0, .0041, .043, .2, .39, .77, 1.54, 2.27, 4.08] * 1e-3 J  mosfet_Erec_data=[0, .0031, .021, .11, .21, .43, .99; 0, .0041, .043, .2, .39, .77, 1.54] * 1e-3 J  gto_Tj_loss=[298.15, 398.15] K  igbt_Tj_loss=[298.15, 398.15] K  mosfet_Tj_loss=[298.15, 398.15] K  gto_Iout_data_loss=[0, .1, 1, 5, 10, 20, 40, 70, 100] A  igbt_Iout_data_loss=[0, .1, 1, 5, 10, 20, 40, 70, 100] A  mosfet_Iout_data_loss=[0, 10, 50, 100, 200, 400, 600] A  gto_Eon_scalar=22.86e-3 J  igbt_Eon_scalar=22.86e-3 J  mosfet_Eon_scalar=22.86e-3 J  gto_Eoff_scalar=17.14e-3 J  igbt_Eoff_scalar=17.14e-3 J  mosfet_Eoff_scalar=17.14e-3 J  gto_Erec_scalar=5.70e-3 J  igbt_Erec_scalar=5.70e-3 J  mosfet_Erec_scalar=5.70e-3 J  gto_Iout_scalar=600 A  igbt_Iout_scalar=600 A  mosfet_Iout_scalar=600 A  igbt_Vce_loss=[0, 150, 300] V  mosfet_Vds_loss=[0, 150, 300] V  Voff=300 V  gtoDiodeErecMat3D=zeros(2, 3, 3) J  igbtDiodeErecMat3D=zeros(2, 3, 3) J  mosfetDiodeErecMat3D=zeros(2, 3, 3) J  gtoTjVecForErec=[298.15, 398.15] K  igbtTjVecForErec=[298.15, 398.15] K  mosfetTjVecForErec=[298.15, 398.15] K  gtoIakVecForErec=[0, 20, 40] A  igbtIceVecForErec=[0, 20, 40] A  mosfetIdsVecForErec=[0, 100, 200] A  gtoVakVecForErec=[0, 150, 300] V  igbtVceVecForErec=[0, 150, 300] V  mosfetVdsVecForErec=[0, 150, 300] V  gto_Eoff_natural_commutation=10e-3 J  applySwLossToSupply=false  tauApplySwLoss=1e-3 s  diode_param=ee.enum.include.yes  diode_ModelType=ee.enum.converters.diodeModelType.pwl  diode_TableType=ee.enum.diode.tableType.IfMat  diode_ReverseIVType=ee.enum.diode.diodeReverseIV.constant  diode_IfMat=[.07, .12, .19, 1.75, 4.24, 7.32, 11.2; .16, .3, .72, 2.14, 4.02, 6.35, 9.12] A  diode_VfMat=[.9, 1.15, 1.25, 1.5, 1.75, 2.17, 2.6, 2.85; .58, .68, .75, 1.1, 1.38, 1.77, 2.27, 2.7] V  diode_TjVec=[25, 125] degC  diode_VfVec=[.5, .7, .9, 1.3, 1.7, 2.1, 2.5] V  diode_IfVec=[.1, .2, .5, 1, 2, 4, 7, 10] A  diode_IrMat=[1e-06, 2e-06, 5e-06, 1e-05, 2.5e-05, 5e-05, .0001; 2e-06, 5e-06, 1e-05, 4e-05, 8e-05, .0002, .0005] A  diode_VrMat=[10, 100, 200, 250, 300, 325, 350; 10, 70, 160, 220, 270, 300, 320] V  diode_VrVec=[10, 20, 40, 50, 70, 80, 100] V  diode_IrVec=[1e-06, 2e-06, 5e-06, 1e-05, 2e-05, 5e-05, .0001] A  diode_Vf=0.8 V  diode_Ron=0.001 Ohm  diode_Goff=1e-5 1/Ohm  separateThermalPort=false  separateThermalPortsForDiodes=false  thermal_network_parameterization=ee.enum.thermalNetworkTopology.external  thermal_mass_parameterization=ee.enum.thermalNetwork.timeconstant  Rth=[.03, .2] K/W  Rth_Cauer=[.03, .1, .2] K/W  Rth_Foster=[.08, .14, .22, .16] K/W  thermal_mass=[3, 25] J/K  thermal_mass_Cauer=[3, 10, 25] J/K  thermal_mass_Foster=[.001, .005, .05, .5] J/K  thermal_time_constant=[.1, 5] s  thermal_time_constant_Cauer=[.1, 1, 5] s  thermal_time_constant_Foster=[7e-05, .0007, .01, .08] s  thermal_mass_initial_temperatures=[25, 25] degC  thermal_mass_initial_temperatures_Cauer=[25, 25, 25] degC  junction_thermal_mass=0.1 J/K  Tvec_initial_Foster=[25, 25, 25, 25] degC  RthDiode=[.03, .2] K/W  RthCauerDiode=[.03, .1, .2] K/W  RthFosterDiode=[.08, .14, .22, .16] K/W  ThermalMassDiode=[3, 25] J/K  ThermalMassCauerDiode=[3, 10, 25] J/K  ThermalMassFosterDiode=[.001, .005, .05, .5] J/K  ThermalTauDiode=[.1, 5] s  ThermalTauCauerDiode=[.1, 1, 5] s  ThermalTauFosterDiode=[7e-05, .0007, .01, .08] s  ThermalMassInitTempDiode=[25, 25] degC  ThermalMassInitTempCauerDiode=[25, 25, 25] degC  JunctionThermalMassDiode=0.1 J/K  TVecInitialFosterDiode=[25, 25, 25, 25] degC  junction_temperature_specify=off  junction_temperature_priority=None  junction_temperature=25 degC  junction_temperature_nominal_specify=off  junction_temperature_nominal_value=1  junction_temperature_nominal_unit=degC  upperSwitchTemp_specify=off  upperSwitchTemp_priority=None  upperSwitchTemp=25 degC  upperSwitchTemp_nominal_specify=off  upperSwitchTemp_nominal_value=1  upperSwitchTemp_nominal_unit=degC  lowerSwitchTemp_specify=off  lowerSwitchTemp_priority=None  lowerSwitchTemp=25 degC  lowerSwitchTemp_nominal_specify=off  lowerSwitchTemp_nominal_value=1  lowerSwitchTemp_nominal_unit=degC  upperDiodeTemp_specify=off  upperDiodeTemp_priority=None  upperDiodeTemp=25 degC  upperDiodeTemp_nominal_specify=off  upperDiodeTemp_nominal_value=1  upperDiodeTemp_nominal_unit=degC  lowerDiodeTemp_specify=off  lowerDiodeTemp_priority=None  lowerDiodeTemp=25 degC  lowerDiodeTemp_nominal_specify=off  lowerDiodeTemp_nominal_value=1  lowerDiodeTemp_nominal_unit=degC
  NOT : Logic  Operator=NOT  IconShape=distinctive  AllPortsSameDT=off  OutDataTypeStr=boolean
  NOT1 : Logic  Operator=NOT  IconShape=distinctive  AllPortsSameDT=off  OutDataTypeStr=boolean
  NOT2 : Logic  Operator=NOT  IconShape=distinctive  AllPortsSameDT=off  OutDataTypeStr=boolean
  PS-Simulink Converter1 : nesl_utility/PS-Simulink Converter  PhysicalDomain=network_engine_domain  SubClassName=ps_output  LeftPortType=input  RightPortType=output  PseudoPeriodic=off  Frequencies=[]  VectorFormat=inherit  Unit=inherit  AffineConversion=off
  PS-Simulink Converter2 : nesl_utility/PS-Simulink Converter  PhysicalDomain=network_engine_domain  SubClassName=ps_output  LeftPortType=input  RightPortType=output  PseudoPeriodic=off  Frequencies=[]  VectorFormat=inherit  Unit=inherit  AffineConversion=off
  PS-Simulink Converter3 : nesl_utility/PS-Simulink Converter  PhysicalDomain=network_engine_domain  SubClassName=ps_output  LeftPortType=input  RightPortType=output  PseudoPeriodic=off  Frequencies=[]  VectorFormat=inherit  Unit=inherit  AffineConversion=off
  Relational Operator : RelationalOperator  Operator=<=  OutDataTypeStr=boolean  RndMeth=Simplest  InputSameDT=off
  Relational Operator1 : RelationalOperator  Operator=<=  OutDataTypeStr=boolean  RndMeth=Simplest  InputSameDT=off
  Relational Operator2 : RelationalOperator  Operator=<=  OutDataTypeStr=boolean  RndMeth=Simplest  InputSameDT=off
  Simulink-PS Converter{,1..3} (4 alike) : nesl_utility/Simulink-PS Converter  PhysicalDomain=network_engine_domain  SubClassName=ps_input  LeftPortType=input  RightPortType=output  PseudoPeriodic=off  Frequencies=[]  NoiseDistribution=none  NoiseParameters=[]  Unit=1  AffineConversion=off  FilteringAndDerivatives=provide  SimscapeFilterOrder=1  InputFilterTimeConstant=0.001  UdotUserProvided=0
  Solver Configuration : nesl_utility/Solver Configuration  PhysicalDomain=network_engine_domain  SubClassName=solver  LeftPortType=input  RightPortType=generic  Tones=[]  Harmonics=[]  SimulateNoise=off  Profile=off  UseLocalSampling=off  EnableSwitchedLinearOptims=on  FrequencyDomain=off  UseCCode=off  RelTol=0.001  AbsTol=0.001  MinStep=1e-09  ToWorkspace=off  RevertToSquareIcSolve=off  NumHomotopyIterations=100  PhasorMode=off  PhasorModeNumHarmonics=1  ConsistencySolver=NEWTON_XTOL_AFTER_FTOL  CanonicalOrdering=UNORDERED  OptimizeIntermediates=UNOPTIMIZED  IndexReductionMethod=DerivativeReplacement  DoDC=off  ResidualTolerance=1e-09  ConsistencyTolSource=GLOBAL  ConsistencyAbsTol=0.001  ConsistencyRelTol=0.001  ConsistencyTolFactor=0.001  UseLocalSolver=off  LocalSolverChoice=NE_BACKWARD_EULER_ADVANCER  ResolveIndetEquations=on  FunctionEvalNumThread=1  LocalSolverSampleTime=0.001  DoFixedCost=off  MaxNonlinIter=3  MaxModeIter=2  ComputeImpulses=off  ImpulseIterations=2  LinearAlgebra=auto  LinearAlgebraNumThread=0  EquationFormulation=NE_TIME_EF  DelaysMemoryBudget=1024  AutomaticFiltering=on  FilteringTimeConstant=0.001  PartitionStorageMethod=AS_NEEDED  PartitionMemoryBudget=1024  PartitionMethod=ROBUST  MultibodyUseLocalSolver=off  MultibodyLocalSolverChoice=ODE1  MultibodyLocalSolverSampleTime=0.001
  Voltage Sensor1 : fl_lib/Electrical/Electrical Sensors/Voltage Sensor
  Voltage Sensor2 : fl_lib/Electrical/Electrical Sensors/Voltage Sensor
  Voltage Sensor3 : fl_lib/Electrical/Electrical Sensors/Voltage Sensor
  Voltage_Output_A : PMIOPort  Side=Right
  Voltage_Output_B : PMIOPort  Port=2  Side=Right
  Voltage_Output_C : PMIOPort  Port=3  Side=Right
  Out1 : Outport
  Out2 : Outport  Port=2
  Out3 : Outport  Port=3
  wires:
  DC_Voltage/1 -> Simulink-PS Converter/1  "DC_Voltage"
  NOT/1 -> Gain2/1
  Relational Operator/1 -> Gain1/1, NOT/1
  Gain2/1 -> Bus Creator2/1
  Gain1/1 -> Bus Creator2/2
  Bus Creator2/1 -> Simulink-PS Converter1/1
  Signal_Carry/1 -> Relational Operator1/2, Relational Operator2/2, Relational Operator/2  "Signal_Carry"
  In2/1 -> Relational Operator/1  "Signal_Radio_A"
  Relational Operator1/1 -> Gain3/1, NOT1/1
  NOT1/1 -> Gain4/1
  Gain4/1 -> Bus Creator1/1
  Bus Creator1/1 -> Simulink-PS Converter2/1
  Gain3/1 -> Bus Creator1/2
  Relational Operator2/1 -> Gain5/1, NOT2/1
  NOT2/1 -> Gain6/1
  Gain6/1 -> Bus Creator3/1
  Bus Creator3/1 -> Simulink-PS Converter3/1
  Gain5/1 -> Bus Creator3/2
  In1/1 -> Relational Operator1/1  "Signal_Radio_B"
  In3/1 -> Relational Operator2/1  "Signal_Radio_C"
  PS-Simulink Converter3/1 -> Out1/1  "Signal_Output_A"
  PS-Simulink Converter2/1 -> Out2/1  "Signal_Output_B"
  PS-Simulink Converter1/1 -> Out3/1  "Signal_Output_C"
  connections:
  Electrical Reference5/LConn1 -- "Half-Bridge (Ideal, Switching)3"/RConn2
  Electrical Reference1/LConn1 -- "Half-Bridge (Ideal, Switching)4"/RConn2
  "Half-Bridge (Ideal, Switching)5"/RConn2 -- Electrical Reference2/LConn1
  "Half-Bridge (Ideal, Switching)3"/LConn3 -- Solver Configuration/RConn1 -- Controlled Voltage Source/LConn1 -- "Half-Bridge (Ideal, Switching)5"/LConn3 -- "Half-Bridge (Ideal, Switching)4"/LConn3
  Electrical Reference3/LConn1 -- Controlled Voltage Source/RConn2
  Simulink-PS Converter/RConn1 -- Controlled Voltage Source/RConn1
  Simulink-PS Converter1/RConn1 -- "Half-Bridge (Ideal, Switching)3"/LConn1
  Simulink-PS Converter2/RConn1 -- "Half-Bridge (Ideal, Switching)4"/LConn1
  Simulink-PS Converter3/RConn1 -- "Half-Bridge (Ideal, Switching)5"/LConn1
  Voltage Sensor3/LConn1 -- Voltage_Output_A/RConn1 -- "Half-Bridge (Ideal, Switching)3"/RConn1
  Voltage Sensor1/LConn1 -- Voltage_Output_B/RConn1 -- "Half-Bridge (Ideal, Switching)4"/RConn1
  Voltage Sensor2/LConn1 -- Voltage_Output_C/RConn1 -- "Half-Bridge (Ideal, Switching)5"/RConn1
  Electrical Reference4/LConn1 -- Voltage Sensor3/RConn2 -- Voltage Sensor1/RConn2 -- Voltage Sensor2/RConn2
  PS-Simulink Converter1/LConn1 -- Voltage Sensor2/RConn1
  PS-Simulink Converter2/LConn1 -- Voltage Sensor1/RConn1
  PS-Simulink Converter3/LConn1 -- Voltage Sensor3/RConn1

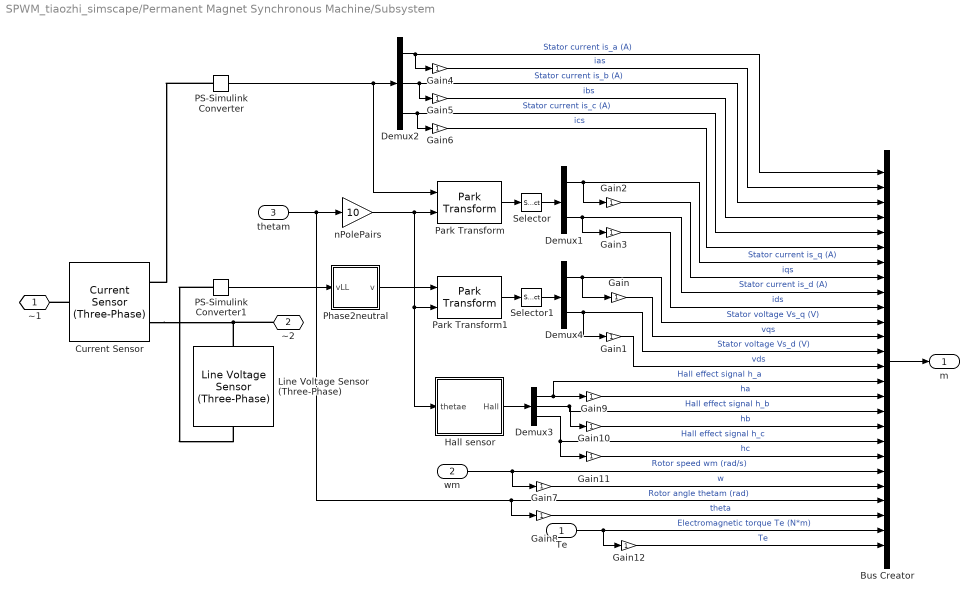
== system SPWM_tiaozhi_simscape/Permanent Magnet Synchronous Machine/Subsystem ==
  Te : Inport
  wm : Inport  Port=2
  thetam : Inport  Port=3
  Bus Creator : BusCreator  Inputs=26
  Current Sensor : ee_lib/Sensors & Transducers/Current Sensor (Three-Phase)  port_option=ee.enum.threePhasePort.composite
  Demux1 : Demux  Outputs=2
  Demux2 : Demux  Outputs=3
  Demux3 : Demux  Outputs=3
  Demux4 : Demux  Outputs=2
  Gain{,1..12} (13 alike) : Gain
  Hall sensor : Subsystem
  Line Voltage Sensor (Three-Phase) : ee_lib/Sensors & Transducers/Line Voltage Sensor (Three-Phase)  port_option=ee.enum.threePhasePort.composite
  PS-Simulink Converter : nesl_utility/PS-Simulink Converter  PhysicalDomain=network_engine_domain  SubClassName=ps_output  LeftPortType=input  RightPortType=output  PseudoPeriodic=off  Frequencies=[]  VectorFormat=1-D array  Unit=1  AffineConversion=off
  PS-Simulink Converter1 : nesl_utility/PS-Simulink Converter  PhysicalDomain=network_engine_domain  SubClassName=ps_output  LeftPortType=input  RightPortType=output  PseudoPeriodic=off  Frequencies=[]  VectorFormat=1-D array  Unit=1  AffineConversion=off
  Park Transform : eeTransforms/Park Transform  AxisAlignment=D-axis  PowerInvariant=off
  Park Transform1 : eeTransforms/Park Transform  AxisAlignment=D-axis  PowerInvariant=off
  Phase2neutral : Subsystem
  Selector : Selector  InputPortWidth=3  IndexOptions=Index vector (dialog)  Indices=[2 1]  OutputSizes=1
  Selector1 : Selector  InputPortWidth=3  IndexOptions=Index vector (dialog)  Indices=[2 1]  OutputSizes=1
  nPolePairs : Gain  Gain=10
  ~1 : PMIOPort  Side=Left
  ~2 : PMIOPort  Port=2  Side=Right
  m : Outport  VectorParamsAs1DForOutWhenUnconnected=off
  wires:
  Phase2neutral/1(v) -> Park Transform1/1
  Gain8/1 -> Bus Creator/24  "theta"
  Gain7/1 -> Bus Creator/22  "w"
  Selector1/1 -> Demux4/1
  Selector/1 -> Demux1/1
  Gain11/1 -> Bus Creator/20  "hc"
  Gain10/1 -> Bus Creator/18  "hb"
  Gain9/1 -> Bus Creator/16  "ha"
  Gain1/1 -> Bus Creator/14  "vds"
  Gain/1 -> Bus Creator/12  "vqs"
  Gain3/1 -> Bus Creator/10  "ids"
  Gain2/1 -> Bus Creator/8  "iqs"
  Hall sensor/1(Hall) -> Demux3/1
  PS-Simulink Converter1/1 -> Phase2neutral/1(vLL)
  Gain6/1 -> Bus Creator/6  "ics"
  Gain5/1 -> Bus Creator/4  "ibs"
  Gain4/1 -> Bus Creator/2  "ias"
  PS-Simulink Converter/1 -> Demux2/1, Park Transform/1
  Te/1 -> Bus Creator/25, Gain12/1  "Electromagnetic torque Te (N*m)"
  Gain12/1 -> Bus Creator/26  "Te"
  Demux3/3 -> Bus Creator/19, Gain11/1  "Hall effect signal h_c"
  Demux3/2 -> Gain10/1, Bus Creator/17  "Hall effect signal h_b"
  Demux3/1 -> Gain9/1, Bus Creator/15  "Hall effect signal h_a"
  thetam/1 -> nPolePairs/1, Gain8/1, Bus Creator/23  "Rotor angle thetam (rad)"
  Bus Creator/1 -> m/1
  Demux2/3 -> Bus Creator/5, Gain6/1  "Stator current is_c (A)"
  Demux2/2 -> Gain5/1, Bus Creator/3  "Stator current is_b (A)"
  Demux2/1 -> Gain4/1, Bus Creator/1  "Stator current is_a (A)"
  Demux1/2 -> Gain3/1, Bus Creator/9  "Stator current is_d (A)"
  Park Transform/1 -> Selector/1
  Demux1/1 -> Gain2/1, Bus Creator/7  "Stator current is_q (A)"
  Demux4/2 -> Gain1/1, Bus Creator/13  "Stator voltage Vs_d (V)"
  Demux4/1 -> Gain/1, Bus Creator/11  "Stator voltage Vs_q (V)"
  Park Transform1/1 -> Selector1/1
  nPolePairs/1 -> Hall sensor/1(thetae), Park Transform1/2, Park Transform/2
  wm/1 -> Bus Creator/21, Gain7/1  "Rotor speed wm (rad/s)"
  connections:
  PS-Simulink Converter1/LConn1 -- Line Voltage Sensor (Three-Phase)/RConn1
  PS-Simulink Converter/LConn1 -- Current Sensor/RConn1
  ~2/RConn1 -- Line Voltage Sensor (Three-Phase)/LConn1 -- Current Sensor/RConn2
  Current Sensor/LConn1 -- ~1/RConn1

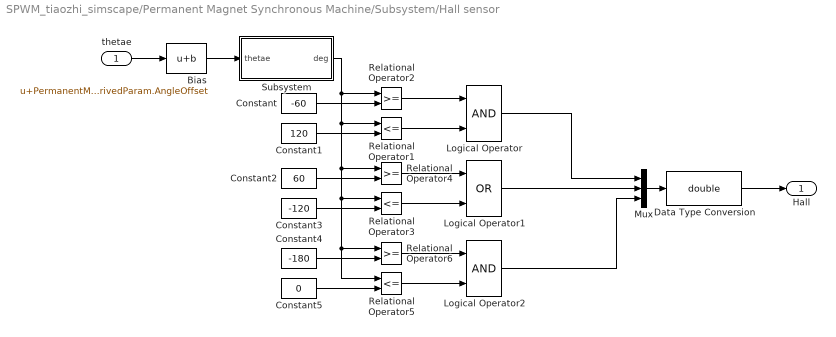
== system SPWM_tiaozhi_simscape/Permanent Magnet Synchronous Machine/Subsystem/Hall sensor ==
  thetae : Inport
  Bias : Bias  Bias=PermanentMagnetSynchrono_class('Torque Tm',[0.00062 0.0003505 10 0],4,'Flux linkage established by magnets (V.s)',0.074147,134.4878,1.1122,'Aligned with phase A axis (original Park)',[0 1 0 0],'Sinusoidal',120,'3',[0 0 0 0 0 0]).objParamMappingDerived.NewDerivedParam.AngleOffset  SaturateOnIntegerOverflow=off
  Constant : Constant  Value=-60
  Constant1 : Constant  Value=120
  Constant2 : Constant  Value=60
  Constant3 : Constant  Value=-120
  Constant4 : Constant  Value=-180
  Constant5 : Constant  Value=0
  Data Type Conversion : DataTypeConversion  OutDataTypeStr=double  SaturateOnIntegerOverflow=off  RndMeth=Floor
  Logical Operator : Logic  AllPortsSameDT=off  OutDataTypeStr=boolean
  Logical Operator1 : Logic  Operator=OR  AllPortsSameDT=off  OutDataTypeStr=boolean
  Logical Operator2 : Logic  AllPortsSameDT=off  OutDataTypeStr=boolean
  Mux : Mux  Inputs=3
  Relational Operator1 : RelationalOperator  Operator=<=
  Relational Operator2 : RelationalOperator
  Relational Operator3 : RelationalOperator  Operator=<=
  Relational Operator4 : RelationalOperator
  Relational Operator5 : RelationalOperator  Operator=<=
  Relational Operator6 : RelationalOperator
  Subsystem : Subsystem
  Hall : Outport  VectorParamsAs1DForOutWhenUnconnected=off
  wires:
  Bias/1 -> Subsystem/1(thetae)
  Data Type Conversion/1 -> Hall/1
  thetae/1 -> Bias/1
  Constant2/1 -> Relational Operator4/2
  Constant1/1 -> Relational Operator1/2
  Relational Operator4/1 -> Logical Operator1/1
  Constant/1 -> Relational Operator2/2
  Subsystem/1(deg) -> Relational Operator2/1, Relational Operator1/1, Relational Operator6/1, Relational Operator5/1, Relational Operator3/1, Relational Operator4/1
  Relational Operator1/1 -> Logical Operator/2
  Relational Operator2/1 -> Logical Operator/1
  Mux/1 -> Data Type Conversion/1
  Relational Operator3/1 -> Logical Operator1/2
  Constant5/1 -> Relational Operator5/2
  Constant4/1 -> Relational Operator6/2
  Relational Operator6/1 -> Logical Operator2/1
  Relational Operator5/1 -> Logical Operator2/2
  Logical Operator/1 -> Mux/1
  Logical Operator1/1 -> Mux/2
  Logical Operator2/1 -> Mux/3
  Constant3/1 -> Relational Operator3/2

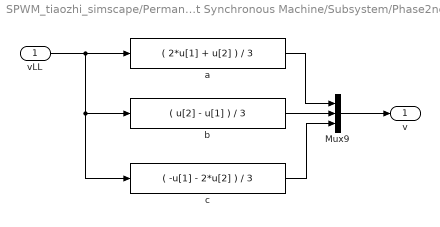
== system SPWM_tiaozhi_simscape/Permanent Magnet Synchronous Machine/Subsystem/Phase2neutral ==
  vLL : Inport
  Mux9 : Mux  Inputs=3
  a : Fcn  Expr=( 2*u[1] + u[2] ) / 3
  b : Fcn  Expr=( u[2] - u[1] ) / 3
  c : Fcn  Expr=( -u[1] - 2*u[2] ) / 3
  v : Outport
  wires:
  b/1 -> Mux9/2
  vLL/1 -> b/1, c/1, a/1
  c/1 -> Mux9/3
  a/1 -> Mux9/1
  Mux9/1 -> v/1

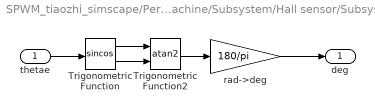
== system SPWM_tiaozhi_simscape/Permanent Magnet Synchronous Machine/Subsystem/Hall sensor/Subsystem ==
  thetae : Inport
  Trigonometric Function : Trigonometry  Operator=sincos
  Trigonometric Function2 : Trigonometry  Operator=atan2
  rad->deg : Gain  Gain=180/pi  SaturateOnIntegerOverflow=on  OutDataTypeStr=Inherit: Same as input  ParamDataTypeStr=Inherit: Same as input
  deg : Outport  VectorParamsAs1DForOutWhenUnconnected=off
  wires:
  thetae/1 -> Trigonometric Function/1
  Trigonometric Function/2 -> Trigonometric Function2/2
  rad->deg/1 -> deg/1
  Trigonometric Function/1 -> Trigonometric Function2/1
  Trigonometric Function2/1 -> rad->deg/1
